simulink model "model"  (R2021a)
settings: Solver=VariableStepAuto  StartTime=0.0  StopTime=2  MaxStep=0.01  RelTol=1e-3
InitFcn:
  | start
model workspace (MAT data in the model file):
  a21 = -3.8563
  a22 = -925.9299
  a31 = 29.0994
  a32 = 121.336777955
  b2 = 1900.51294583
  b3 = -249.049215835
values from neighbouring files (symbols this model uses):
  A = [0 0 1 ... (first row only)    [matrix_set.m]
  B = [0 ... (first row only)    [matrix_set.m]
  K = lqr(A,B,QQ,RR)    [matrix_set.m]
  Psi0 = pi/12    (= 0.261799387799)    [start_config.m]
  Psi_d0 = 0    [start_config.m]
  Theta_d0 = 0    [start_config.m]
  Umax = 8.2    [variables_set.m]
settings Model: PauseTimes=1  SnapshotBufferSize=8000  Creator=danii  LastModifiedBy=Dmitry
settings SolverCC: ZeroCrossAlgorithm=Adaptive  AlgebraicLoopSolver=TrustRegion
settings DataIOCC: ReturnWorkspaceOutputs=off
settings DebuggingCC: SFMachineParentedDataDiag=warning  ArithmeticOperatorsInVariantConditions=warning
settings SFSimCC: SimUseLocalCustomCode=off  CustomCodeUndefinedFunction=UseInterfaceOnly
settings RTWCC: RTWUseLocalCustomCode=off
settings CodeAppCC: StateflowObjectComments=on
settings ConfigComp: PSAutoStubLUT=on

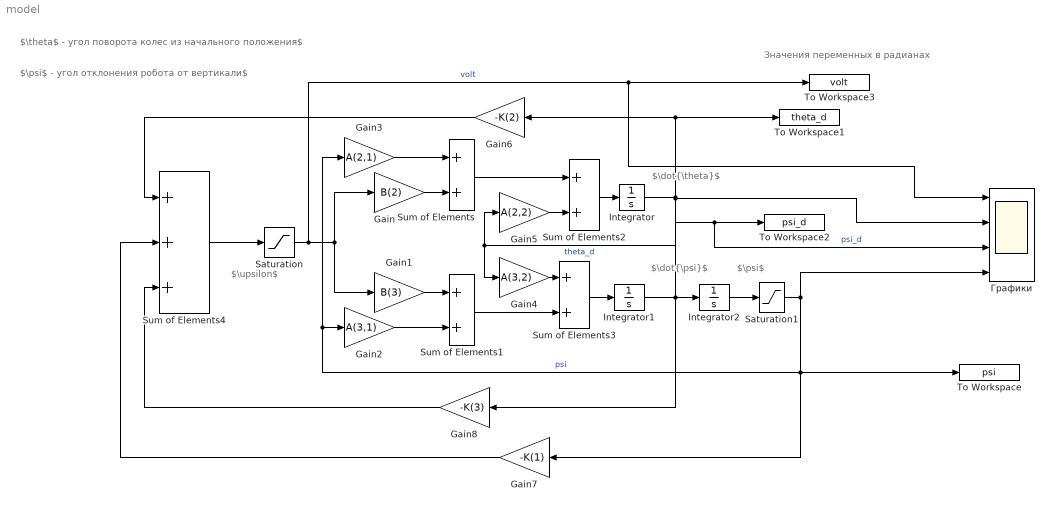
== system model ==
  note: $\dot{\theta}$
  note: Значения переменных в радианах
  note: $\dot{\psi}$
  note: $\psi$
  note: $\theta$ - угол поворота колес из начального положения$
  note: $\psi$ - угол отклонения робота от вертикали$
  note: $\upsilon$
  Gain : Gain  Gain=B(2)
  Gain1 : Gain  Gain=B(3)
  Gain2 : Gain  Gain=A(3,1)
  Gain3 : Gain  Gain=A(2,1)
  Gain4 : Gain  Gain=A(3,2)
  Gain5 : Gain  Gain=A(2,2)
  Gain6 : Gain  Gain=-K(2)
  Gain7 : Gain  Gain=-K(1)
  Gain8 : Gain  Gain=-K(3)
  Integrator : Integrator  InitialCondition=Theta_d0
  Integrator1 : Integrator  InitialCondition=Psi_d0
  Integrator2 : Integrator  InitialCondition=Psi0
  Saturation : Saturate  UpperLimit=Umax  LowerLimit=-Umax
  Saturation1 : Saturate  UpperLimit=pi/180*95  LowerLimit=-pi/180*95
  Sum of Elements{,1..3} (4 alike) : Sum  Inputs=2
  Sum of Elements4 : Sum  Inputs=3
  To Workspace : ToWorkspace  VariableName=psi  SampleTime=-1
  To Workspace1 : ToWorkspace  VariableName=theta_d  SampleTime=-1
  To Workspace2 : ToWorkspace  VariableName=psi_d  SampleTime=-1
  To Workspace3 : ToWorkspace  VariableName=volt  SampleTime=-1
  Графики : Scope  NumInputPorts=4
  wires:
  Saturation/1 -> Графики/1, To Workspace3/1, Gain1/1, Gain/1  "volt"
  Gain/1 -> Sum of Elements/2
  Gain1/1 -> Sum of Elements1/1
  Gain2/1 -> Sum of Elements1/2
  Gain3/1 -> Sum of Elements/1
  Sum of Elements/1 -> Sum of Elements2/1
  Sum of Elements1/1 -> Sum of Elements3/2
  Gain5/1 -> Sum of Elements2/2
  Gain4/1 -> Sum of Elements3/1
  Sum of Elements2/1 -> Integrator/1
  Sum of Elements3/1 -> Integrator1/1
  Integrator/1 -> Gain4/1, Gain5/1, Графики/2, To Workspace1/1, Gain6/1  "theta_d"
  Integrator1/1 -> Gain8/1, To Workspace2/1, Графики/3, Integrator2/1  "psi_d"
  Sum of Elements4/1 -> Saturation/1
  Gain7/1 -> Sum of Elements4/2
  Gain8/1 -> Sum of Elements4/3
  Integrator2/1 -> Saturation1/1
  Gain6/1 -> Sum of Elements4/1
  Saturation1/1 -> To Workspace/1, Gain7/1, Gain3/1, Gain2/1, Графики/4  "psi"
